simulink model "rural_tele_triage"  (R2026a)
settings: Solver=VariableStepAuto

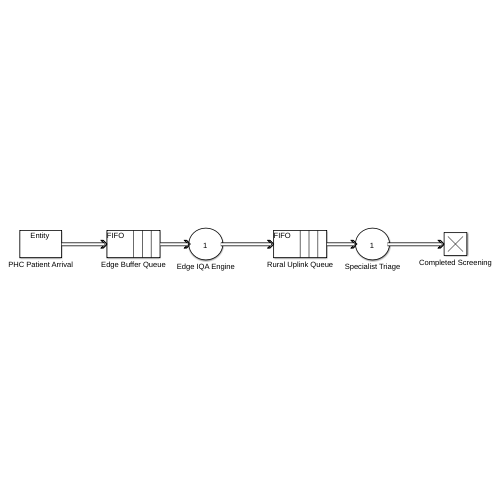
[thumbnail: Simulink's stored preview of the top-level diagram]
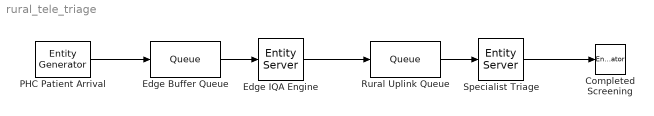
== system rural_tele_triage ==
  Completed Screening : EntityTerminator  InputPortMessageModes=m
  Edge Buffer Queue : Queue  InputPortMessageModes=m  OutputPortMessageModes=m
  Edge IQA Engine : EntityServer  InputPortMessageModes=m  OutputPortMessageModes=m  Capacity=1
  PHC Patient Arrival : EntityGenerator  OutputPortMessageModes=m  EntityType=Structured  EntityTypeName=Entity
  Rural Uplink Queue : Queue  InputPortMessageModes=m  OutputPortMessageModes=m
  Specialist Triage : EntityServer  InputPortMessageModes=m  OutputPortMessageModes=m  Capacity=1
  wires:
  Specialist Triage/1 -> Completed Screening/1
  Rural Uplink Queue/1 -> Specialist Triage/1
  Edge IQA Engine/1 -> Rural Uplink Queue/1
  Edge Buffer Queue/1 -> Edge IQA Engine/1
  PHC Patient Arrival/1 -> Edge Buffer Queue/1
